simulink model "Takeoff_Sim"  (R2023a)
settings: Solver=VariableStepAuto  StartTime=0.0  StopTime=35  RelTol=1e-3
values from neighbouring files (symbols this model uses):
  AoA = 5    [initialize.m]
  AR = 6.4897    [initialize.m]
  f = 6.271    [initialize.m]
  S = 174    [initialize.m]
  Weight = 2518    [initialize.m]
undefined symbols (not defined in the file or in its folder): Accelerometer, Accelerometerdeland, Earth, Gyroscope, Gyroscopedeland, Location, Locationdeland, WGS84
libraries: simulink_extras x10, aerolibtransform2 x4, simulink x4, aerolibatmos2 x2
(part 1 of 2)
settings Model: Creator=NAILSK  LastModifiedBy=kaleb
settings RTWCC: GPUComputeCapability=5.0

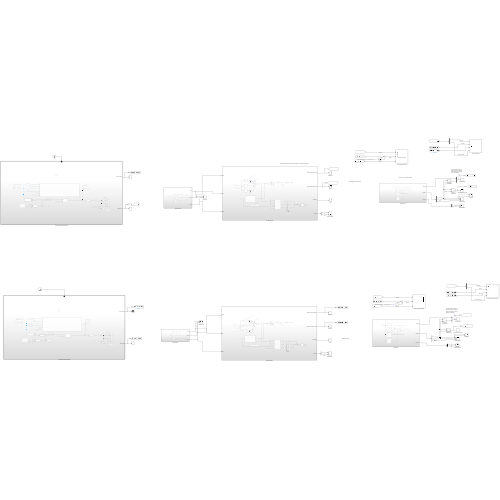
[thumbnail: Simulink's stored preview of the top-level diagram]
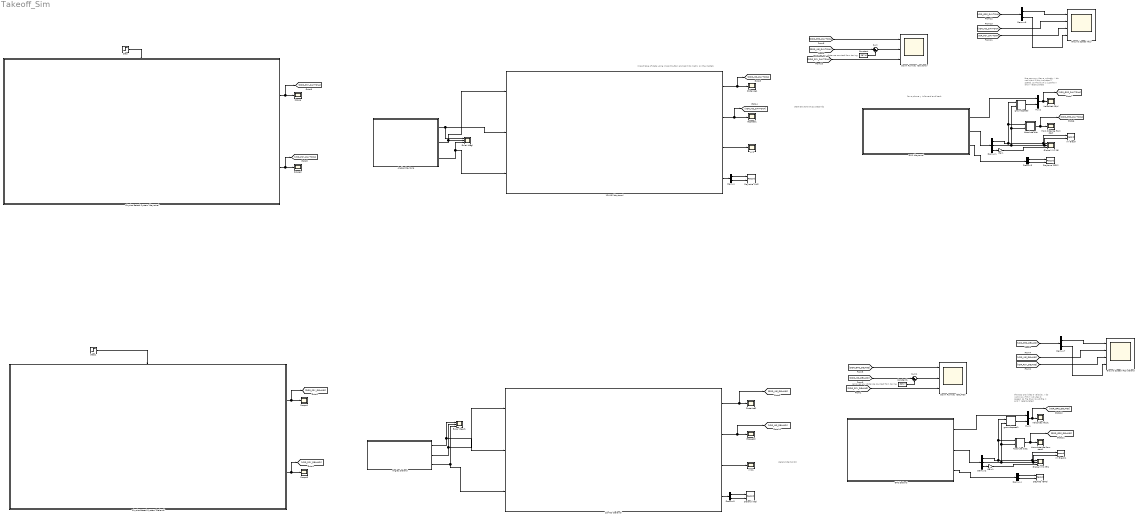
== system Takeoff_Sim ==
  note: removes any distance counted from taxing
  note: deland start at 20
  note: Start Daytona at 22 Seconds
  note: the app provides a velocity, I do not know if this includes Z speed, so the blue is just the X and Y recalculated
  note: for a phone y is foward and back
  note: import take of data using import button and set it to matrix on the matlab
  note: the app provides a velocity, I do not know if this includes Z speed, so the blue is just the X and Y recalculated
  note: removes any distance counted from taxing
  1D-INS (Deland) : Subsystem
  1D-INS (daytona) : Subsystem
  Absolute dist : Subsystem
  Absolute dist1 : Subsystem
  Angles Daytona : Subsystem
  Angles Deland : Subsystem
  Constant : Constant  Value=287.6
  Constant1 : Constant  Value=509.7
  DELAND (GPS) : Record  FileSettingsInternal="{\"entries\":[{\"content\":{\"excelSettings\":{\"content\":{},\"type\":\"Streamout.ExcelSettings\"}},\"type\":\"Streamout.FileSettingStorage\",\"uuid\":\"\"}],\"packageUris\":[\"http:\\/\\/schema.mathworks.com\\/mf0\\/streamout_blocks\\/R2020a\"],\"version\":\"1.0\"}"  Layout=[1 1]  SignalsInternal="{\"entries\":[{\"content\":{\"signals\":[{\"content\":{\"blockPath\":[],\"dimensions\":[1],\"domain\":\"\",\"lineColor\":\"#77ac30\",\"plots\":[1],\"port\":1,\"sid\":[\"\"],\"signalID\":63633,\"signalName\":\"Lat\"},\"type\":\"RecordBlkView.Signal\",\"uuid\":\"\"},{\"content\":{\"blockPath\":[],\"dimensions\":[1],\"domain\":\"\",\"lineColor\":\"#4dbeee\",\"plots\":[1],\"port\":2,\"sid\":[\"\"],\"signalID\":63637,\"signalName\":\"Long\"},\"type\":\"RecordBlkView.Signal\",\"uuid\":\"\"}]},\"type\":\"RecordBlkView.InputSignals\",\"uuid\":\"\"}],\"packageUris\":[\"http:\\/\\/schema.mathworks.com\\/mf0\\/streamout_blocks\\/R2020a\"],\"version\":\"1.0\"}"  VisualizationBindings="{\"mapsplugin\":{\"info\":[{\"bindingParametersList\":[{\"parameter\":\"Latitude\",\"signalID\":63633,\"signalName\":\"Lat\"},{\"parameter\":\"Longitude\",\"signalID\":63637,\"signalName\":\"Long\"}],\"subplotID\":1}]}}"  CompatibilityTag=XY
  Daytona (GPS) : Record  FileSettingsInternal="{\"entries\":[{\"content\":{\"excelSettings\":{\"content\":{},\"type\":\"Streamout.ExcelSettings\"}},\"type\":\"Streamout.FileSettingStorage\",\"uuid\":\"\"}],\"packageUris\":[\"http:\\/\\/schema.mathworks.com\\/mf0\\/streamout_blocks\\/R2020a\"],\"version\":\"1.0\"}"  Layout=[1 1]  SignalsInternal="{\"entries\":[{\"content\":{\"signals\":[{\"content\":{\"blockPath\":[],\"dimensions\":[1],\"domain\":\"\",\"lineColor\":\"#0072bd\",\"plots\":[1],\"port\":1,\"sid\":[\"\"],\"signalID\":63657,\"signalName\":\"Lat\"},\"type\":\"RecordBlkView.Signal\",\"uuid\":\"\"},{\"content\":{\"blockPath\":[],\"dimensions\":[1],\"domain\":\"\",\"lineColor\":\"#d95319\",\"plots\":[1],\"port\":2,\"sid\":[\"\"],\"signalID\":63661,\"signalName\":\"Long\"},\"type\":\"RecordBlkView.Signal\",\"uuid\":\"\"}]},\"type\":\"RecordBlkView.InputSignals\",\"uuid\":\"\"}],\"packageUris\":[\"http:\\/\\/schema.mathworks.com\\/mf0\\/streamout_blocks\\/R2020a\"],\"version\":\"1.0\"}"  VisualizationBindings="{\"mapsplugin\":{\"info\":[{\"bindingParametersList\":[{\"parameter\":\"Latitude\",\"signalID\":63657,\"signalName\":\"Lat\"},{\"parameter\":\"Longitude\",\"signalID\":63661,\"signalName\":\"Long\"}],\"subplotID\":1}]}}"  CompatibilityTag=XY
  Daytona (INS) : Record  FileSettingsInternal="{\"entries\":[{\"content\":{\"excelSettings\":{\"content\":{},\"type\":\"Streamout.ExcelSettings\"}},\"type\":\"Streamout.FileSettingStorage\",\"uuid\":\"\"}],\"packageUris\":[\"http:\\/\\/schema.mathworks.com\\/mf0\\/streamout_blocks\\/R2020a\"],\"version\":\"1.0\"}"  Layout=[1 1]  SignalsInternal="{\"entries\":[{\"content\":{\"signals\":[{\"content\":{\"blockPath\":[],\"dimensions\":[1],\"domain\":\"\",\"lineColor\":\"#a2142f\",\"plots\":[1],\"port\":1,\"sid\":[\"\"],\"signalID\":63665,\"signalName\":\"Lat\"},\"type\":\"RecordBlkView.Signal\",\"uuid\":\"\"},{\"content\":{\"blockPath\":[],\"dimensions\":[1],\"domain\":\"\",\"lineColor\":\"#139fff\",\"plots\":[1],\"port\":2,\"sid\":[\"\"],\"signalID\":63669,\"signalName\":\"Long\"},\"type\":\"RecordBlkView.Signal\",\"uuid\":\"\"}]},\"type\":\"RecordBlkView.InputSignals\",\"uuid\":\"\"}],\"packageUris\":[\"http:\\/\\/schema.mathworks.com\\/mf0\\/streamout_blocks\\/R2020a\"],\"version\":\"1.0\"}"  VisualizationBindings="{\"mapsplugin\":{\"info\":[{\"bindingParametersList\":[{\"parameter\":\"Latitude\",\"signalID\":63665,\"signalName\":\"Lat\"},{\"parameter\":\"Longitude\",\"signalID\":63669,\"signalName\":\"Long\"}],\"subplotID\":1}]}}"  CompatibilityTag=XY
  Deland (INS) : Record  FileSettingsInternal="{\"entries\":[{\"content\":{\"excelSettings\":{\"content\":{},\"type\":\"Streamout.ExcelSettings\"}},\"type\":\"Streamout.FileSettingStorage\",\"uuid\":\"\"}],\"packageUris\":[\"http:\\/\\/schema.mathworks.com\\/mf0\\/streamout_blocks\\/R2020a\"],\"version\":\"1.0\"}"  Layout=[1 1]  SignalsInternal="{\"entries\":[{\"content\":{\"signals\":[{\"content\":{\"blockPath\":[],\"dimensions\":[1],\"domain\":\"\",\"lineColor\":\"#ff6929\",\"plots\":[1],\"port\":1,\"sid\":[\"\"],\"signalID\":63641,\"signalName\":\"Lat\"},\"type\":\"RecordBlkView.Signal\",\"uuid\":\"\"},{\"content\":{\"blockPath\":[],\"dimensions\":[1],\"domain\":\"\",\"lineColor\":\"#b746ff\",\"plots\":[1],\"port\":2,\"sid\":[\"\"],\"signalID\":63645,\"signalName\":\"Long\"},\"type\":\"RecordBlkView.Signal\",\"uuid\":\"\"}]},\"type\":\"RecordBlkView.InputSignals\",\"uuid\":\"\"}],\"packageUris\":[\"http:\\/\\/schema.mathworks.com\\/mf0\\/streamout_blocks\\/R2020a\"],\"version\":\"1.0\"}"  VisualizationBindings="{\"mapsplugin\":{\"info\":[{\"bindingParametersList\":[{\"parameter\":\"Latitude\",\"signalID\":63641,\"signalName\":\"Lat\"},{\"parameter\":\"Longitude\",\"signalID\":63645,\"signalName\":\"Long\"}],\"subplotID\":1}]}}"  CompatibilityTag=XY
  Demux{,3..7} (6 alike) : Demux  Outputs=2
  Demux1 : Demux  Outputs=3
  Demux2 : Demux  Outputs=3
  Distance1 : Scope
  Distance2 : Scope
  Down Runway (DELAND) : Scope  NumInputPorts=3
  Down Runway (Daytona) : Scope  NumInputPorts=3
  Euler (deg) : Scope  NumInputPorts=3
  Euler (deg)1 : Scope  NumInputPorts=3
  GPS (daytona) : Subsystem
  GPS Deland : Subsystem
  Gain : Gain  Gain=-1
  Gain1 : Gain  Gain=-1
  Global XYZ (ft) : Scope  NumInputPorts=3
  Global XYZ (ft)1 : Scope  NumInputPorts=3
  Ground Speed (ft/s) : Scope  NumInputPorts=4
  Ground Speed (ft/s) deland : Scope  NumInputPorts=4
  Gspeed1 : Scope
  Gspeed2 : Scope
  Horz distance from start : Scope
  Horz distance from start1 : Scope
  Mux1 : Mux  Inputs=2
  Mux2 : Mux  Inputs=2
  Physics Based System (Deland) : Subsystem  TreatAsAtomicUnit=on
  Physics Based System (daytona) : Subsystem  TreatAsAtomicUnit=on
  Scope{,1..3} (4 alike) : Scope
  Step : Step  Time=22  SampleTime=0
  Step1 : Step  Time=20  SampleTime=0
  Sum : Sum  Inputs=|+-
  Sum1 : Sum  Inputs=|+-
  Velocities (ft/s) : Scope
  Velocities (ft/s)1 : Scope
  XY Graph : Record  FileSettingsInternal="{\"entries\":[{\"content\":{\"excelSettings\":{\"content\":{},\"type\":\"Streamout.ExcelSettings\"}},\"type\":\"Streamout.FileSettingStorage\",\"uuid\":\"\"}],\"packageUris\":[\"http:\\/\\/schema.mathworks.com\\/mf0\\/streamout_blocks\\/R2020a\"],\"version\":\"1.0\"}"  Layout=[1 1]  SignalsInternal="{\"entries\":[{\"content\":{\"signals\":[{\"content\":{\"blockPath\":[],\"dimensions\":[1],\"domain\":\"\",\"lineColor\":\"#a2142f\",\"plots\":[1],\"port\":1,\"sid\":[\"\"],\"signalID\":63673,\"signalName\":\"x\"},\"type\":\"RecordBlkView.Signal\",\"uuid\":\"\"},{\"content\":{\"blockPath\":[],\"dimensions\":[1],\"domain\":\"\",\"lineColor\":\"#139fff\",\"plots\":[1],\"port\":2,\"sid\":[\"\"],\"signalID\":63677,\"signalName\":\"y\"},\"type\":\"RecordBlkView.Signal\",\"uuid\":\"\"}]},\"type\":\"RecordBlkView.InputSignals\",\"uuid\":\"\"}],\"packageUris\":[\"http:\\/\\/schema.mathworks.com\\/mf0\\/streamout_blocks\\/R2020a\"],\"version\":\"1.0\"}"  VisualizationBindings="{\"xyplotplugin\":{\"info\":[{\"series\":[{\"bindingParametersList\":[{\"parameter\":\"X-Axis\",\"signalID\":63673,\"signalName\":\"x\"},{\"parameter\":\"Y-Axis\",\"signalID\":63677,\"signalName\":\"y\"}],\"seriesID\":32496}],\"subplotID\":1}]}}"  CompatibilityTag=XY
  XY Graph1 : Record  FileSettingsInternal="{\"entries\":[{\"content\":{\"excelSettings\":{\"content\":{},\"type\":\"Streamout.ExcelSettings\"}},\"type\":\"Streamout.FileSettingStorage\",\"uuid\":\"\"}],\"packageUris\":[\"http:\\/\\/schema.mathworks.com\\/mf0\\/streamout_blocks\\/R2020a\"],\"version\":\"1.0\"}"  Layout=[1 1]  SignalsInternal="{\"entries\":[{\"content\":{\"signals\":[{\"content\":{\"blockPath\":[],\"dimensions\":[1],\"domain\":\"\",\"lineColor\":\"#a2142f\",\"plots\":[1],\"port\":1,\"sid\":[\"\"],\"signalID\":63649,\"signalName\":\"x\"},\"type\":\"RecordBlkView.Signal\",\"uuid\":\"\"},{\"content\":{\"blockPath\":[],\"dimensions\":[1],\"domain\":\"\",\"lineColor\":\"#139fff\",\"plots\":[1],\"port\":2,\"sid\":[\"\"],\"signalID\":63653,\"signalName\":\"y\"},\"type\":\"RecordBlkView.Signal\",\"uuid\":\"\"}]},\"type\":\"RecordBlkView.InputSignals\",\"uuid\":\"\"}],\"packageUris\":[\"http:\\/\\/schema.mathworks.com\\/mf0\\/streamout_blocks\\/R2020a\"],\"version\":\"1.0\"}"  VisualizationBindings="{\"xyplotplugin\":{\"info\":[{\"series\":[{\"bindingParametersList\":[{\"parameter\":\"X-Axis\",\"signalID\":63649,\"signalName\":\"x\"},{\"parameter\":\"Y-Axis\",\"signalID\":63653,\"signalName\":\"y\"}],\"seriesID\":5620}],\"subplotID\":1}]}}"  CompatibilityTag=XY
  XYZ : Scope
  XYZ1 : Scope
  groundspeed : Subsystem
  groundspeed1 : Subsystem
  wires:
  1D-INS (daytona)/1(Distance Down Runway (ft)) -> [DDR_INS_DAYTONA], Distance1/1
  1D-INS (daytona)/2(Velocity Down Runway (ft/s)) -> [VDR_INS_DAYTONA], Gspeed1/1
  GPS (daytona)/1(velocity) -> Mux2/1
  GPS (daytona)/2(Distance) -> Demux1/1
  Demux1/1 -> Absolute dist/1(x), groundspeed/1(x), XY Graph/1, Global XYZ (ft)/1  "x"
  Demux1/2 -> Absolute dist/2(y), groundspeed/2(y), XY Graph/2, Global XYZ (ft)/2  "y"
  Demux1/3 -> Gain/1  "z"
  Gain/1 -> Global XYZ (ft)/3
  groundspeed/1(Out1) -> Mux2/2
  Mux2/1 -> [VDR_GPS_DAYTONA], Velocities (ft/s)/1
  Angles Daytona/1(roll1) -> 1D-INS (daytona)/2(roll), Euler (deg)/1
  Angles Daytona/2(pitch1) -> 1D-INS (daytona)/1(pitch), Euler (deg)/2
  Angles Daytona/3(yaw1) -> 1D-INS (daytona)/3(yaw), Euler (deg)/3
  Absolute dist/1(Out1) -> [DDR_GPS_DAYTONA], Horz distance from start/1
  1D-INS (daytona)/3(Global (ft/s)) -> XYZ/1
  1D-INS (daytona)/4(Lat/Long) -> Demux/1
  Demux/1 -> Daytona (INS)/1  "Lat"
  Demux/2 -> Daytona (INS)/2  "Long"
  Demux3/1 -> Daytona (GPS)/1  "Lat"
  Demux3/2 -> Daytona (GPS)/2  "Long"
  GPS (daytona)/3(Lat/Long) -> Demux3/1
  Demux5/2 -> Deland (INS)/2  "Long"
  1D-INS (Deland)/3(Global (ft/s)) -> XYZ1/1
  Demux5/1 -> Deland (INS)/1  "Lat"
  1D-INS (Deland)/4(Lat/Long) -> Demux5/1
  1D-INS (Deland)/2(Velocity Down Runway (ft/s)) -> [VDR_INS_DELAND], Gspeed2/1
  1D-INS (Deland)/1(Distance Down Runway (ft)) -> [DDR_INS_DELAND], Distance2/1
  Angles Deland/3(yaw1) -> 1D-INS (Deland)/3(yaw), Euler (deg)1/3
  Angles Deland/2(pitch1) -> Euler (deg)1/2, 1D-INS (Deland)/1(pitch)
  Angles Deland/1(roll1) -> Euler (deg)1/1, 1D-INS (Deland)/2(roll)
  Step/1 -> Physics Based System (daytona)/Enable
  Physics Based System (daytona)/2(Velocity (ft/s)) -> [VDR_PSY_DAYTONA], Scope2/1
  Physics Based System (daytona)/1(Ft down runway) -> [DDR_PSY_DAYTONA], Scope/1
  [DDR_GPS_DAYTONA] -> Down Runway (Daytona)/1  "GPS (ft)"
  [DDR_INS_DAYTONA] -> Sum/1  "INS (ft)"
  [DDR_PSY_DAYTONA] -> Down Runway (Daytona)/3  "PSY (ft)"
  Constant/1 -> Sum/2
  Sum/1 -> Down Runway (Daytona)/2  "INS (ft)"
  [VDR_PSY_DAYTONA] -> Ground Speed (ft/s)/3  "PSY (ft/s)"
  [VDR_INS_DAYTONA] -> Ground Speed (ft/s)/2  "INS (ft/s)"
  [VDR_GPS_DAYTONA] -> Demux6/1
  Demux6/2 -> Ground Speed (ft/s)/4  "Derived GPS (ft/s)"
  Demux6/1 -> Ground Speed (ft/s)/1  "GPS (ft/s)"
  Physics Based System (Deland)/1(Ft down runway) -> Scope1/1, [DDR_PSY_DELAND]
  Physics Based System (Deland)/2(Velocity (ft/s)) -> Scope3/1, [VDR_PSY_DELAND]
  Step1/1 -> Physics Based System (Deland)/Enable
  groundspeed1/1(Out1) -> Mux1/2
  Absolute dist1/1(Out1) -> [DDR_GPS_DELAND], Horz distance from start1/1
  Demux4/2 -> DELAND (GPS)/2  "Long"
  GPS Deland/1(velocity) -> Mux1/1
  Gain1/1 -> Global XYZ (ft)1/3
  GPS Deland/3(Lat/Long) -> Demux4/1
  Demux2/1 -> Absolute dist1/1(x), groundspeed1/1(x), XY Graph1/1, Global XYZ (ft)1/1  "x"
  GPS Deland/2(Distance) -> Demux2/1
  Demux2/3 -> Gain1/1  "z"
  Demux4/1 -> DELAND (GPS)/1  "Lat"
  Mux1/1 -> [VDR_GPS_DELAND], Velocities (ft/s)1/1
  Demux2/2 -> Absolute dist1/2(y), groundspeed1/2(y), XY Graph1/2, Global XYZ (ft)1/2  "y"
  Demux7/1 -> Ground Speed (ft/s) deland/1  "GPS (ft/s)"
  Demux7/2 -> Ground Speed (ft/s) deland/4  "Derived GPS (ft/s)"
  [VDR_GPS_DELAND] -> Demux7/1
  [VDR_INS_DELAND] -> Ground Speed (ft/s) deland/2  "INS (ft/s)"
  [VDR_PSY_DELAND] -> Ground Speed (ft/s) deland/3  "PSY (ft/s)"
  Sum1/1 -> Down Runway (DELAND)/2  "INS (ft)"
  Constant1/1 -> Sum1/2
  [DDR_PSY_DELAND] -> Down Runway (DELAND)/3  "PSY (ft)"
  [DDR_INS_DELAND] -> Sum1/1  "INS (ft)"
  [DDR_GPS_DELAND] -> Down Runway (DELAND)/1  "GPS (ft)"

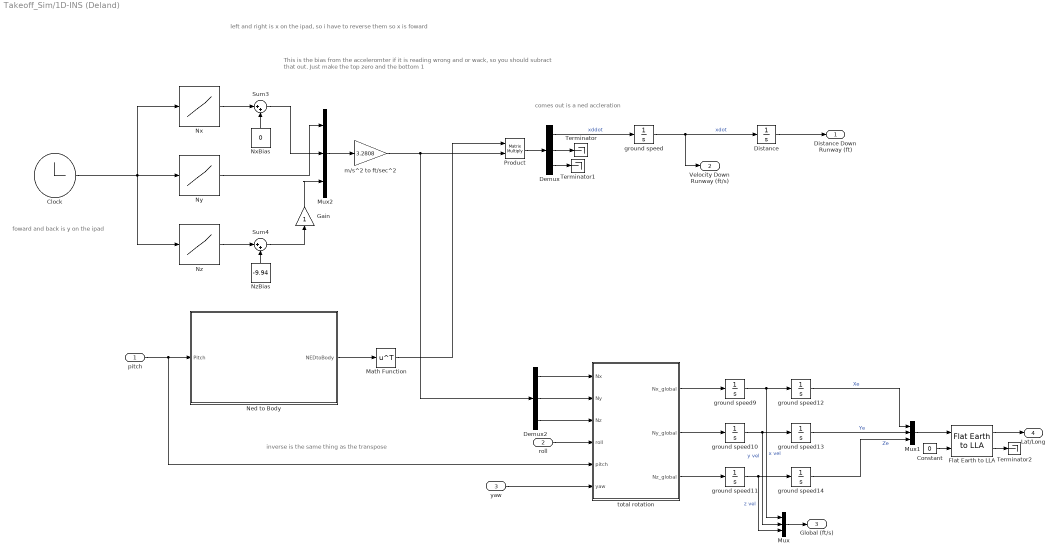
== system Takeoff_Sim/1D-INS (Deland) ==
  note: foward and back is y on the ipad
  note: left and right is x on the ipad, so i have to reverse them so x is foward
  note: This is the bias from the acceleromter if it is reading wrong and or wack, so you should subract that out. Just make the top zero and the bottom 1
  note: inverse is the same thing as the transpose
  note: comes out is a ned accleration
  pitch : Inport
  roll : Inport  Port=2
  yaw : Inport  Port=3
  Clock : Clock
  Constant : Constant  Value=0
  Demux : Demux  Outputs=3
  Demux2 : Demux  Outputs=3
  Distance : Integrator
  Flat Earth to LLA : aerolibtransform2/Flat Earth to LLA  units=English  ptype=Earth (WGS84)  F=1/298.257223563  R=20925646.3255  refPosPort=off  LL0=[2.906098674E1 -8.128727349E1]  psi=0
  Gain : Gain
  Math Function : Math  Operator=transpose
  Mux : Mux  Inputs=3
  Mux1 : Mux  Inputs=3
  Mux2 : Mux  Inputs=3
  Ned to Body : Subsystem
  Nx : Lookup_n-D  NumberOfTableDimensions=1  BreakpointsForDimension1=Accelerometerdeland(:,1)  Table=Accelerometerdeland(:,2)  InternalRulePriority=Speed  RndMeth=Simplest
  NxBias : Constant  Value=0
  Ny : Lookup_n-D  NumberOfTableDimensions=1  BreakpointsForDimension1=Accelerometerdeland(:,1)  Table=Accelerometerdeland(:,3)  InternalRulePriority=Speed  RndMeth=Simplest
  Nz : Lookup_n-D  NumberOfTableDimensions=1  BreakpointsForDimension1=Accelerometerdeland(:,1)  Table=Accelerometerdeland(:,4)  InternalRulePriority=Speed  RndMeth=Simplest
  NzBias : Constant  Value=-9.94
  Product : Product  Multiplication=Matrix(*)
  Sum3 : Sum  Inputs=|++
  Sum4 : Sum  Inputs=|++
  Terminator : Terminator
  Terminator1 : Terminator
  Terminator2 : Terminator
  ground speed : Integrator  InitialCondition=8.55
  ground speed{9..14} (6 alike) : Integrator
  m/s^2 to ft/sec^2 : Gain  Gain=3.2808
  total rotation : MATLAB Function  TreatAsAtomicUnit=on
  Distance Down Runway (ft) : Outport
  Velocity Down Runway (ft/s) : Outport  Port=2
  Global (ft/s) : Outport  Port=3
  Lat/Long : Outport  Port=4
  wires:
  Sum3/1 -> Mux2/2
  Product/1 -> Demux/1
  Ned to Body/1(NEDtoBody) -> Math Function/1
  Nz/1 -> Sum4/1
  Clock/1 -> Nx/1, Nz/1, Ny/1
  Mux2/1 -> m/s^2 to ft/sec^2/1
  NxBias/1 -> Sum3/2
  Nx/1 -> Sum3/1
  NzBias/1 -> Sum4/2
  m/s^2 to ft/sec^2/1 -> Demux2/1, Product/2
  Demux/1 -> ground speed/1  "xddot"
  Math Function/1 -> Product/1
  ground speed/1 -> Distance/1, Velocity Down Runway (ft/s)/1  "xdot"
  Ny/1 -> Mux2/1
  Sum4/1 -> Gain/1
  Distance/1 -> Distance Down Runway (ft)/1
  pitch/1 -> total rotation/5(pitch), Ned to Body/1(Pitch)
  Demux2/1 -> total rotation/1(Nx)
  Demux2/2 -> total rotation/2(Ny)
  Demux2/3 -> total rotation/3(Nz)
  roll/1 -> total rotation/4(roll)
  ground speed14/1 -> Mux1/3  "Ze"
  ground speed13/1 -> Mux1/2  "Ye"
  ground speed12/1 -> Mux1/1  "Xe"
  ground speed11/1 -> Mux/3, ground speed14/1  "z vel"
  ground speed10/1 -> Mux/2, ground speed13/1  "y vel"
  ground speed9/1 -> Mux/1, ground speed12/1  "x vel"
  total rotation/3(Nz_global) -> ground speed11/1
  total rotation/2(Ny_global) -> ground speed10/1
  total rotation/1(Nx_global) -> ground speed9/1
  Demux/2 -> Terminator/1
  Demux/3 -> Terminator1/1
  Mux/1 -> Global (ft/s)/1
  Constant/1 -> Flat Earth to LLA/2
  Flat Earth to LLA/2 -> Terminator2/1
  Mux1/1 -> Flat Earth to LLA/1
  Flat Earth to LLA/1 -> Lat/Long/1
  yaw/1 -> total rotation/6(yaw)
  Gain/1 -> Mux2/3

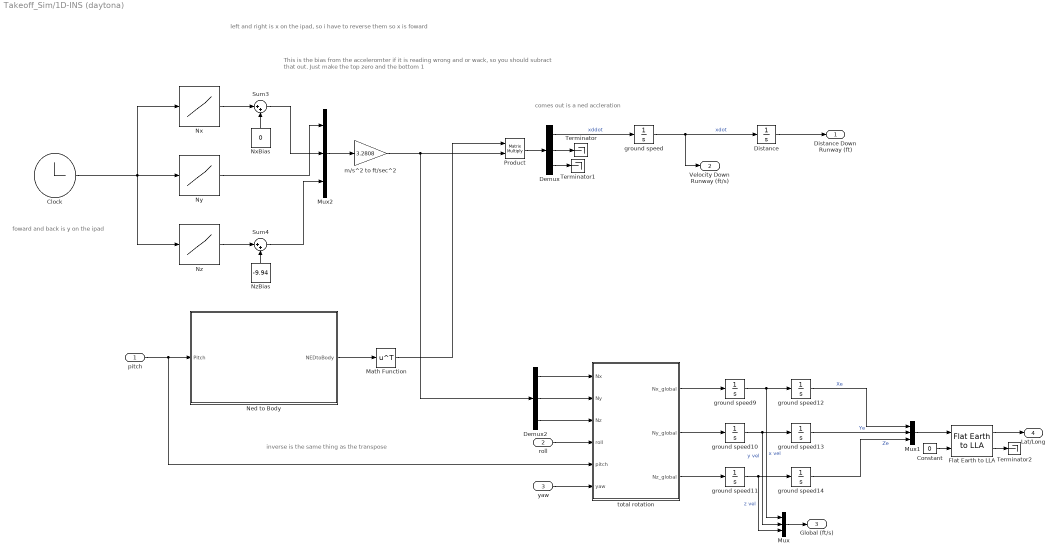
== system Takeoff_Sim/1D-INS (daytona) ==
  note: foward and back is y on the ipad
  note: left and right is x on the ipad, so i have to reverse them so x is foward
  note: This is the bias from the acceleromter if it is reading wrong and or wack, so you should subract that out. Just make the top zero and the bottom 1
  note: inverse is the same thing as the transpose
  note: comes out is a ned accleration
  pitch : Inport
  roll : Inport  Port=2
  yaw : Inport  Port=3
  Clock : Clock
  Constant : Constant  Value=0
  Demux : Demux  Outputs=3
  Demux2 : Demux  Outputs=3
  Distance : Integrator
  Flat Earth to LLA : aerolibtransform2/Flat Earth to LLA  units=English  ptype=Earth (WGS84)  F=1/298.257223563  R=20925646.3255  refPosPort=off  LL0=[2.917987119E1 -8.106194666E1]  psi=0
  Math Function : Math  Operator=transpose
  Mux : Mux  Inputs=3
  Mux1 : Mux  Inputs=3
  Mux2 : Mux  Inputs=3
  Ned to Body : Subsystem
  Nx : Lookup_n-D  NumberOfTableDimensions=1  BreakpointsForDimension1=Accelerometer(:,1)  Table=Accelerometer(:,2)  InternalRulePriority=Speed  RndMeth=Simplest
  NxBias : Constant  Value=0
  Ny : Lookup_n-D  NumberOfTableDimensions=1  BreakpointsForDimension1=Accelerometer(:,1)  Table=Accelerometer(:,3)  InternalRulePriority=Speed  RndMeth=Simplest
  Nz : Lookup_n-D  NumberOfTableDimensions=1  BreakpointsForDimension1=Accelerometer(:,1)  Table=Accelerometer(:,4)  InternalRulePriority=Speed  RndMeth=Simplest
  NzBias : Constant  Value=-9.94
  Product : Product  Multiplication=Matrix(*)
  Sum3 : Sum  Inputs=|++
  Sum4 : Sum  Inputs=|++
  Terminator : Terminator
  Terminator1 : Terminator
  Terminator2 : Terminator
  ground speed{,9..14} (7 alike) : Integrator
  m/s^2 to ft/sec^2 : Gain  Gain=3.2808
  total rotation : MATLAB Function  TreatAsAtomicUnit=on
  Distance Down Runway (ft) : Outport
  Velocity Down Runway (ft/s) : Outport  Port=2
  Global (ft/s) : Outport  Port=3
  Lat/Long : Outport  Port=4
  wires:
  Sum3/1 -> Mux2/2
  Product/1 -> Demux/1
  Ned to Body/1(NEDtoBody) -> Math Function/1
  Nz/1 -> Sum4/1
  Clock/1 -> Nx/1, Nz/1, Ny/1
  Mux2/1 -> m/s^2 to ft/sec^2/1
  NxBias/1 -> Sum3/2
  Nx/1 -> Sum3/1
  NzBias/1 -> Sum4/2
  m/s^2 to ft/sec^2/1 -> Demux2/1, Product/2
  Demux/1 -> ground speed/1  "xddot"
  Math Function/1 -> Product/1
  ground speed/1 -> Distance/1, Velocity Down Runway (ft/s)/1  "xdot"
  Ny/1 -> Mux2/1
  Sum4/1 -> Mux2/3
  Distance/1 -> Distance Down Runway (ft)/1
  pitch/1 -> total rotation/5(pitch), Ned to Body/1(Pitch)
  Demux2/1 -> total rotation/1(Nx)
  Demux2/2 -> total rotation/2(Ny)
  Demux2/3 -> total rotation/3(Nz)
  yaw/1 -> total rotation/6(yaw)
  roll/1 -> total rotation/4(roll)
  ground speed14/1 -> Mux1/3  "Ze"
  ground speed13/1 -> Mux1/2  "Ye"
  ground speed12/1 -> Mux1/1  "Xe"
  ground speed11/1 -> Mux/3, ground speed14/1  "z vel"
  ground speed10/1 -> Mux/2, ground speed13/1  "y vel"
  ground speed9/1 -> Mux/1, ground speed12/1  "x vel"
  total rotation/3(Nz_global) -> ground speed11/1
  total rotation/2(Ny_global) -> ground speed10/1
  total rotation/1(Nx_global) -> ground speed9/1
  Demux/2 -> Terminator/1
  Demux/3 -> Terminator1/1
  Mux/1 -> Global (ft/s)/1
  Constant/1 -> Flat Earth to LLA/2
  Flat Earth to LLA/2 -> Terminator2/1
  Mux1/1 -> Flat Earth to LLA/1
  Flat Earth to LLA/1 -> Lat/Long/1

== system Takeoff_Sim/Absolute dist ==
  note: since this is GPS, i cannot measure from the start, i geo synced this position with a time. because the current data set includes some taxiing , this removes that
  x : Inport
  y : Inport  Port=2
  Abs : Abs  SaturateOnIntegerOverflow=off
  Abs1 : Abs  SaturateOnIntegerOverflow=off
  Start Posx : Constant  Value=-210.4
  Sum : Sum  Inputs=|-+
  Sum1 : Sum  Inputs=|-+
  Sum4 : Sum  Inputs=|++
  start pos y : Constant  Value=164.6
  Out1 : Outport
  wires:
  y/1 -> Sum1/2
  Abs/1 -> Sum4/1
  x/1 -> Sum/2
  Abs1/1 -> Sum4/2
  Sum4/1 -> Out1/1
  Start Posx/1 -> Sum/1
  Sum/1 -> Abs/1
  start pos y/1 -> Sum1/1
  Sum1/1 -> Abs1/1

== system Takeoff_Sim/Absolute dist1 ==
  note: since this is GPS, i cannot measure from the start, i geo synced this position with a time. because the current data set includes some taxiing , this removes that
  x : Inport
  y : Inport  Port=2
  Abs : Abs  SaturateOnIntegerOverflow=off
  Abs1 : Abs  SaturateOnIntegerOverflow=off
  Start Posx : Constant  Value=84.1
  Sum : Sum  Inputs=|-+
  Sum1 : Sum  Inputs=|-+
  Sum4 : Sum  Inputs=|++
  start pos y : Constant  Value=-134.8
  Out1 : Outport
  wires:
  y/1 -> Sum1/2
  Abs/1 -> Sum4/1
  x/1 -> Sum/2
  Abs1/1 -> Sum4/2
  Sum4/1 -> Out1/1
  Start Posx/1 -> Sum/1
  Sum/1 -> Abs/1
  start pos y/1 -> Sum1/1
  Sum1/1 -> Abs1/1

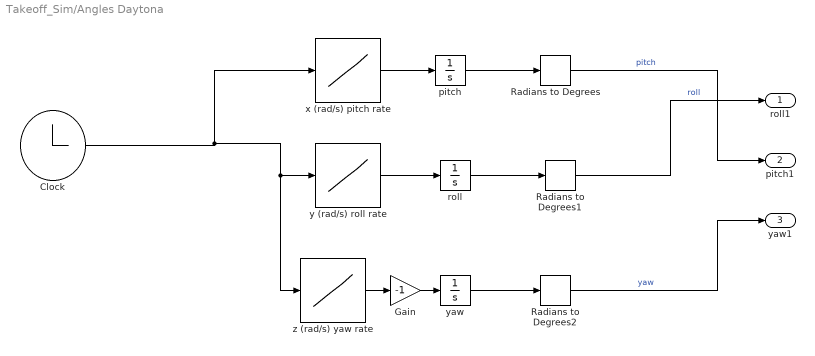
== system Takeoff_Sim/Angles Daytona ==
  Clock : Clock
  Gain : Gain  Gain=-1
  Radians to Degrees : simulink_extras/Transformations/Radians to Degrees
  Radians to Degrees1 : simulink_extras/Transformations/Radians to Degrees
  Radians to Degrees2 : simulink_extras/Transformations/Radians to Degrees
  pitch : Integrator  InitialCondition=.0995
  roll : Integrator
  x (rad/s) pitch rate : Lookup_n-D  NumberOfTableDimensions=1  BreakpointsForDimension1=Gyroscope(:,1)  Table=Gyroscope(:,2)  InternalRulePriority=Speed  RndMeth=Simplest
  y (rad/s) roll rate : Lookup_n-D  NumberOfTableDimensions=1  BreakpointsForDimension1=Gyroscope(:,1)  Table=Gyroscope(:,3)  InternalRulePriority=Speed  RndMeth=Simplest
  yaw : Integrator  InitialCondition=pi/180*165
  z (rad/s) yaw rate : Lookup_n-D  NumberOfTableDimensions=1  BreakpointsForDimension1=Gyroscope(:,1)  Table=Gyroscope(:,4)  InternalRulePriority=Speed  RndMeth=Simplest
  roll1 : Outport
  pitch1 : Outport  Port=2
  yaw1 : Outport  Port=3
  wires:
  pitch/1 -> Radians to Degrees/1
  Radians to Degrees2/1 -> yaw1/1  "yaw"
  yaw/1 -> Radians to Degrees2/1
  Clock/1 -> z (rad/s) yaw rate/1, y (rad/s) roll rate/1, x (rad/s) pitch rate/1
  y (rad/s) roll rate/1 -> roll/1
  roll/1 -> Radians to Degrees1/1
  x (rad/s) pitch rate/1 -> pitch/1
  Radians to Degrees/1 -> pitch1/1  "pitch"
  Radians to Degrees1/1 -> roll1/1  "roll"
  z (rad/s) yaw rate/1 -> Gain/1
  Gain/1 -> yaw/1

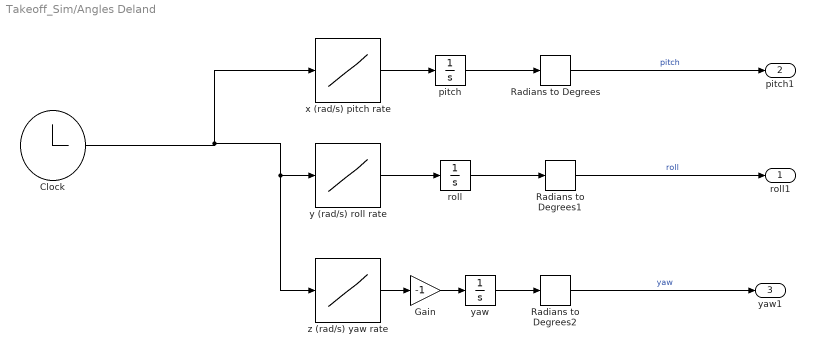
== system Takeoff_Sim/Angles Deland ==
  Clock : Clock
  Gain : Gain  Gain=-1
  Radians to Degrees : simulink_extras/Transformations/Radians to Degrees
  Radians to Degrees1 : simulink_extras/Transformations/Radians to Degrees
  Radians to Degrees2 : simulink_extras/Transformations/Radians to Degrees
  pitch : Integrator  InitialCondition=.0995
  roll : Integrator
  x (rad/s) pitch rate : Lookup_n-D  NumberOfTableDimensions=1  BreakpointsForDimension1=Gyroscopedeland(:,1)  Table=Gyroscopedeland(:,2)  InternalRulePriority=Speed  RndMeth=Simplest
  y (rad/s) roll rate : Lookup_n-D  NumberOfTableDimensions=1  BreakpointsForDimension1=Gyroscopedeland(:,1)  Table=Gyroscopedeland(:,3)  InternalRulePriority=Speed  RndMeth=Simplest
  yaw : Integrator  InitialCondition=-1.75
  z (rad/s) yaw rate : Lookup_n-D  NumberOfTableDimensions=1  BreakpointsForDimension1=Gyroscopedeland(:,1)  Table=Gyroscopedeland(:,4)  InternalRulePriority=Speed  RndMeth=Simplest
  roll1 : Outport
  pitch1 : Outport  Port=2
  yaw1 : Outport  Port=3
  wires:
  pitch/1 -> Radians to Degrees/1
  Radians to Degrees2/1 -> yaw1/1  "yaw"
  yaw/1 -> Radians to Degrees2/1
  Clock/1 -> z (rad/s) yaw rate/1, y (rad/s) roll rate/1, x (rad/s) pitch rate/1
  y (rad/s) roll rate/1 -> roll/1
  z (rad/s) yaw rate/1 -> Gain/1
  roll/1 -> Radians to Degrees1/1
  x (rad/s) pitch rate/1 -> pitch/1
  Radians to Degrees/1 -> pitch1/1  "pitch"
  Radians to Degrees1/1 -> roll1/1  "roll"
  Gain/1 -> yaw/1

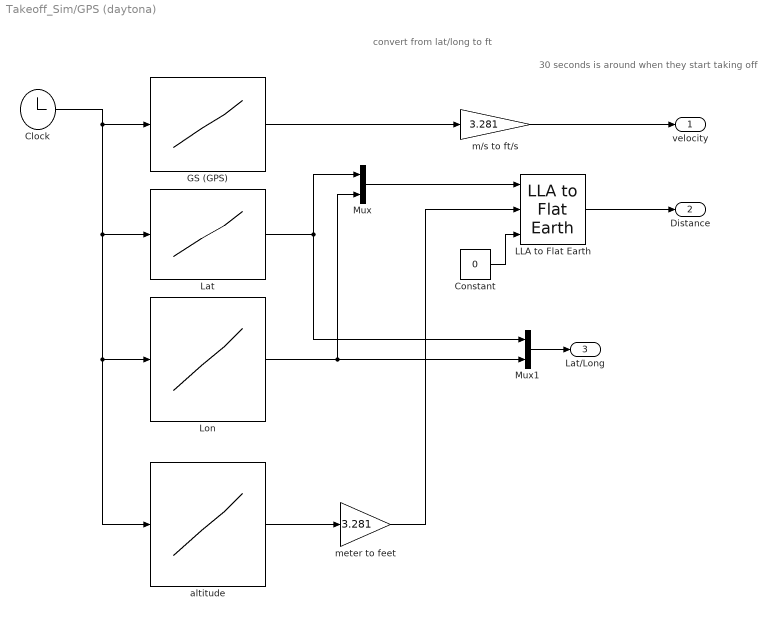
== system Takeoff_Sim/GPS (daytona) ==
  note: 30 seconds is around when they start taking off
  note: convert from lat/long to ft
  Clock : Clock
  Constant : Constant  Value=0
  GS (GPS) : Lookup_n-D  NumberOfTableDimensions=1  BreakpointsForDimension1=Location(:,1)  Table=Location(:,5)  InternalRulePriority=Speed  RndMeth=Simplest
  LLA to Flat Earth : aerolibtransform2/LLA to Flat Earth  units=English  ptype=Earth (WGS84)  F=1/298.257223563  R=20925646.3255  refPosPort=off  LL0=[2.917987119E1 -8.106194666E1]  psi=0
  Lat : Lookup_n-D  NumberOfTableDimensions=1  BreakpointsForDimension1=Location(:,1)  Table=Location(:,2)  InternalRulePriority=Speed  RndMeth=Simplest
  Lon : Lookup_n-D  NumberOfTableDimensions=1  BreakpointsForDimension1=Location(:,1)  Table=Location(:,3)  InternalRulePriority=Speed  RndMeth=Simplest
  Mux : Mux  Inputs=2
  Mux1 : Mux  Inputs=2
  altitude : Lookup_n-D  NumberOfTableDimensions=1  BreakpointsForDimension1=Location(:,1)  Table=Location(:,4)  InternalRulePriority=Speed  RndMeth=Simplest
  m/s to ft/s : Gain  Gain=3.281
  meter to feet : Gain  Gain=3.281
  velocity : Outport
  Distance : Outport  Port=2
  Lat/Long : Outport  Port=3
  wires:
  Clock/1 -> altitude/1, Lon/1, Lat/1, GS (GPS)/1
  Lat/1 -> Mux1/1, Mux/1
  Lon/1 -> Mux/2, Mux1/2
  Mux/1 -> LLA to Flat Earth/1
  GS (GPS)/1 -> m/s to ft/s/1
  m/s to ft/s/1 -> velocity/1
  Constant/1 -> LLA to Flat Earth/3
  altitude/1 -> meter to feet/1
  meter to feet/1 -> LLA to Flat Earth/2
  LLA to Flat Earth/1 -> Distance/1
  Mux1/1 -> Lat/Long/1

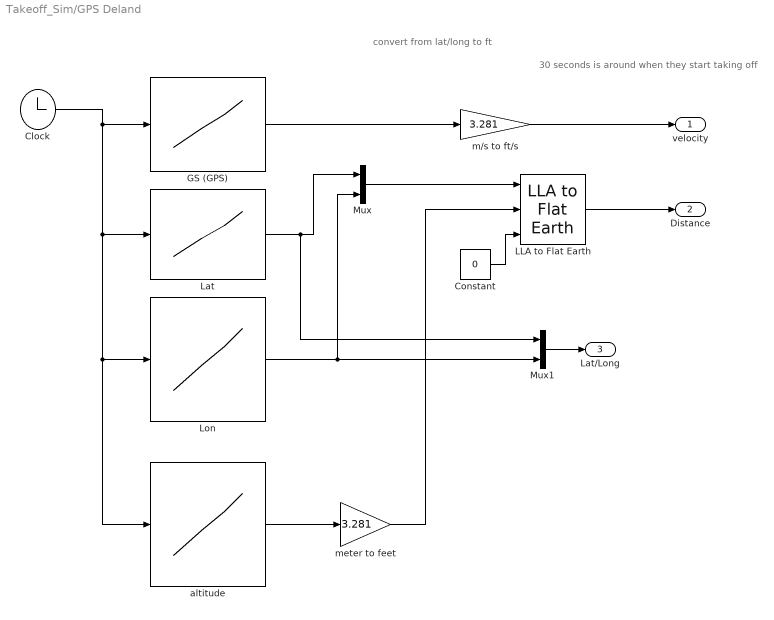
== system Takeoff_Sim/GPS Deland ==
  note: 30 seconds is around when they start taking off
  note: convert from lat/long to ft
  Clock : Clock
  Constant : Constant  Value=0
  GS (GPS) : Lookup_n-D  NumberOfTableDimensions=1  BreakpointsForDimension1=Locationdeland(:,1)  Table=Locationdeland(:,5)  InternalRulePriority=Speed  RndMeth=Simplest
  LLA to Flat Earth : aerolibtransform2/LLA to Flat Earth  units=English  ptype=Earth (WGS84)  F=1/298.257223563  R=20925646.3255  refPosPort=off  LL0=[2.906098674E1 -8.128727349E1]  psi=0
  Lat : Lookup_n-D  NumberOfTableDimensions=1  BreakpointsForDimension1=Locationdeland(:,1)  Table=Locationdeland(:,2)  InternalRulePriority=Speed  RndMeth=Simplest
  Lon : Lookup_n-D  NumberOfTableDimensions=1  BreakpointsForDimension1=Locationdeland(:,1)  Table=Locationdeland(:,3)  InternalRulePriority=Speed  RndMeth=Simplest
  Mux : Mux  Inputs=2
  Mux1 : Mux  Inputs=2
  altitude : Lookup_n-D  NumberOfTableDimensions=1  BreakpointsForDimension1=Locationdeland(:,1)  Table=Locationdeland(:,4)  InternalRulePriority=Speed  RndMeth=Simplest
  m/s to ft/s : Gain  Gain=3.281
  meter to feet : Gain  Gain=3.281
  velocity : Outport
  Distance : Outport  Port=2
  Lat/Long : Outport  Port=3
  wires:
  Clock/1 -> altitude/1, Lon/1, Lat/1, GS (GPS)/1
  Lat/1 -> Mux1/1, Mux/1
  Lon/1 -> Mux/2, Mux1/2
  Mux/1 -> LLA to Flat Earth/1
  GS (GPS)/1 -> m/s to ft/s/1
  m/s to ft/s/1 -> velocity/1
  Constant/1 -> LLA to Flat Earth/3
  altitude/1 -> meter to feet/1
  meter to feet/1 -> LLA to Flat Earth/2
  LLA to Flat Earth/1 -> Distance/1
  Mux1/1 -> Lat/Long/1

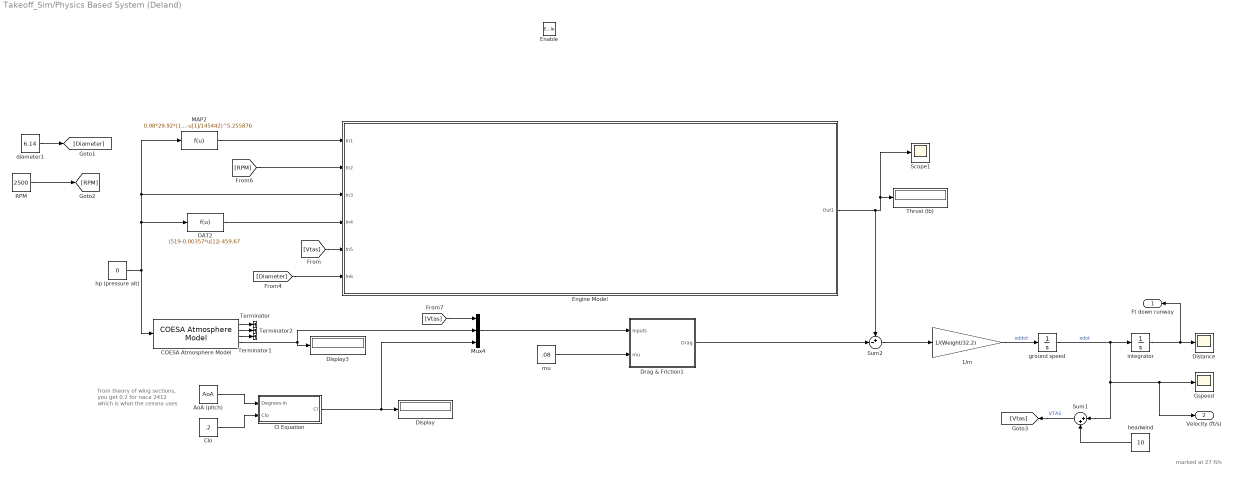
== system Takeoff_Sim/Physics Based System (Deland) ==
  note: from theory of wing sections, you get 0.2 for naca 2412 which is what the cessna uses
  note: marked at 27 ft/s
  Enable : EnablePort
  1/m : Gain  Gain=1/(Weight/32.2)
  AoA (pitch) : Constant  Value=AoA
  COESA Atmosphere Model : aerolibatmos2/COESA Atmosphere Model  units=English (Velocity in ft/s)  spec=1976 COESA-extended U.S. Standard Atmosphere  model=Profile  profile_var=High temperature  profile_percent=1%  profile_alt=5 km (16404 ft)  envelope_var=High temperature  envelope_percent=1%  action=Warning
  Cl Equation : Subsystem
  Clo : Constant  Value=.2
  Display : Display
  Display3 : Display
  Distance : Scope
  Drag & Friction1 : Subsystem  VariantControl=Choice
  Engine Model : Subsystem
  Gspeed : Scope
  MAP2 : Fcn  Expr=0.98*29.92*(1-u[1]/145442)^5.255876
  Mux4 : Mux  Inputs=3
  OAT2 : Fcn  Expr=(519-0.00357*u[1])-459.67
  RPM : Constant  Value=2500
  Scope1 : Scope
  Sum1 : Sum  Inputs=|++
  Sum2 : Sum  Inputs=+-|
  Terminator : Terminator
  Terminator1 : Terminator
  Terminator2 : Terminator
  Thrust (lb) : Display
  diameter1 : Constant  Value=6.14
  ground speed : Integrator  InitialCondition=20
  headwind : Constant  Value=10
  hp (pressure alt) : Constant  Value=0
  integrator : Integrator
  mu : Constant  Value=.08
  Ft down runway : Outport
  Velocity (ft/s) : Outport  Port=2
  wires:
  integrator/1 -> Distance/1, Ft down runway/1
  diameter1/1 -> [Diameter]
  [RPM] -> Engine Model/2(In2)
  OAT2/1 -> Engine Model/4(In4)
  COESA Atmosphere Model/4 -> Mux4/2, Display3/1
  headwind/1 -> Sum1/2
  [Diameter] -> Engine Model/6(In6)
  MAP2/1 -> Engine Model/1(In1)
  hp (pressure alt)/1 -> COESA Atmosphere Model/1, Engine Model/3(In3), MAP2/1, OAT2/1
  ground speed/1 -> integrator/1, Gspeed/1, Velocity (ft/s)/1, Sum1/1  "xdot"
  RPM/1 -> [RPM]
  Mux4/1 -> Drag & Friction1/1(Inputs)
  Cl Equation/1(Cl) -> Display/1, Mux4/3
  1/m/1 -> ground speed/1  "xddot"
  Engine Model/1(Out1) -> Sum2/1, Thrust (lb)/1, Scope1/1
  Sum2/1 -> 1/m/1
  [Vtas] -> Engine Model/5(In5)
  COESA Atmosphere Model/2 -> Terminator2/1
  COESA Atmosphere Model/1 -> Terminator/1
  COESA Atmosphere Model/3 -> Terminator1/1
  AoA (pitch)/1 -> Cl Equation/1(Degrees in)
  Sum1/1 -> [Vtas]  "VTAS"
  mu/1 -> Drag & Friction1/2(mu)
  Drag & Friction1/1(Drag) -> Sum2/2
  Clo/1 -> Cl Equation/2(Clo)
  [Vtas] -> Mux4/1

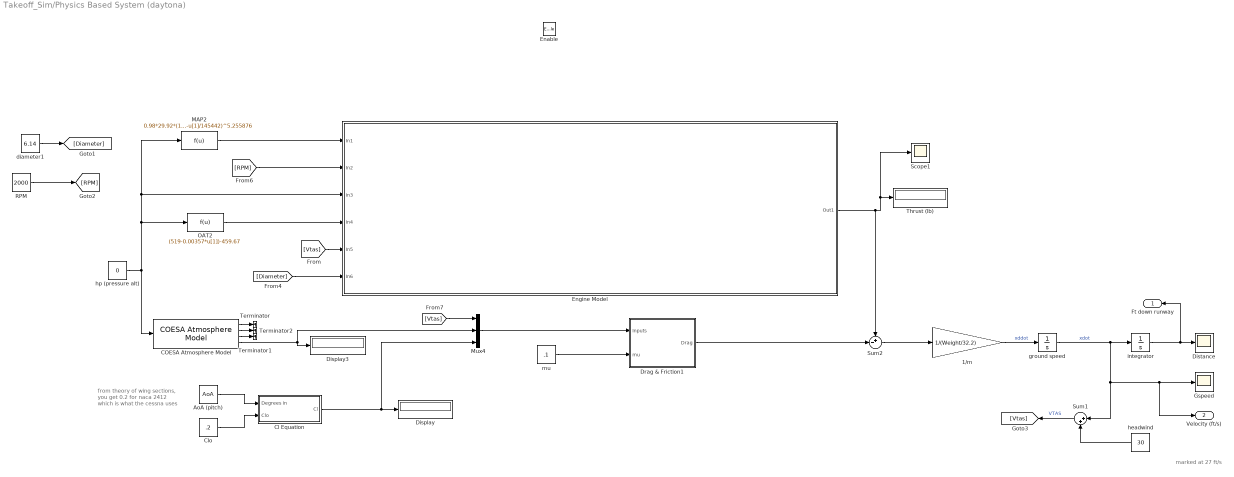
== system Takeoff_Sim/Physics Based System (daytona) ==
  note: marked at 27 ft/s
  note: from theory of wing sections, you get 0.2 for naca 2412 which is what the cessna uses
  Enable : EnablePort
  1/m : Gain  Gain=1/(Weight/32.2)
  AoA (pitch) : Constant  Value=AoA
  COESA Atmosphere Model : aerolibatmos2/COESA Atmosphere Model  units=English (Velocity in ft/s)  spec=1976 COESA-extended U.S. Standard Atmosphere  model=Profile  profile_var=High temperature  profile_percent=1%  profile_alt=5 km (16404 ft)  envelope_var=High temperature  envelope_percent=1%  action=Warning
  Cl Equation : Subsystem
  Clo : Constant  Value=.2
  Display : Display
  Display3 : Display
  Distance : Scope
  Drag & Friction1 : Subsystem  VariantControl=Choice
  Engine Model : Subsystem
  Gspeed : Scope
  MAP2 : Fcn  Expr=0.98*29.92*(1-u[1]/145442)^5.255876
  Mux4 : Mux  Inputs=3
  OAT2 : Fcn  Expr=(519-0.00357*u[1])-459.67
  RPM : Constant  Value=2000
  Scope1 : Scope
  Sum1 : Sum  Inputs=|++
  Sum2 : Sum  Inputs=+-|
  Terminator : Terminator
  Terminator1 : Terminator
  Terminator2 : Terminator
  Thrust (lb) : Display
  diameter1 : Constant  Value=6.14
  ground speed : Integrator  InitialCondition=20
  headwind : Constant  Value=30
  hp (pressure alt) : Constant  Value=0
  integrator : Integrator
  mu : Constant  Value=.1
  Ft down runway : Outport
  Velocity (ft/s) : Outport  Port=2
  wires:
  [Vtas] -> Mux4/1
  Clo/1 -> Cl Equation/2(Clo)
  Drag & Friction1/1(Drag) -> Sum2/2
  mu/1 -> Drag & Friction1/2(mu)
  Sum1/1 -> [Vtas]  "VTAS"
  AoA (pitch)/1 -> Cl Equation/1(Degrees in)
  COESA Atmosphere Model/3 -> Terminator1/1
  COESA Atmosphere Model/1 -> Terminator/1
  COESA Atmosphere Model/2 -> Terminator2/1
  [Vtas] -> Engine Model/5(In5)
  Sum2/1 -> 1/m/1
  Engine Model/1(Out1) -> Scope1/1, Thrust (lb)/1, Sum2/1
  1/m/1 -> ground speed/1  "xddot"
  Cl Equation/1(Cl) -> Mux4/3, Display/1
  Mux4/1 -> Drag & Friction1/1(Inputs)
  RPM/1 -> [RPM]
  ground speed/1 -> Sum1/1, Velocity (ft/s)/1, Gspeed/1, integrator/1  "xdot"
  hp (pressure alt)/1 -> OAT2/1, MAP2/1, Engine Model/3(In3), COESA Atmosphere Model/1
  MAP2/1 -> Engine Model/1(In1)
  [Diameter] -> Engine Model/6(In6)
  headwind/1 -> Sum1/2
  COESA Atmosphere Model/4 -> Display3/1, Mux4/2
  OAT2/1 -> Engine Model/4(In4)
  [RPM] -> Engine Model/2(In2)
  diameter1/1 -> [Diameter]
  integrator/1 -> Ft down runway/1, Distance/1

== system Takeoff_Sim/groundspeed ==
  x : Inport
  y : Inport  Port=2
  Discrete Derivative : simulink/Discrete/Discrete Derivative  gainval=1.0  ICPrevScaledInput=0.0  OutMin=[]  OutMax=[]  OutDataType=fixdt(1, 16)  OutScaling=2^-10  DoSatur=off
  Discrete Derivative1 : simulink/Discrete/Discrete Derivative  gainval=1.0  ICPrevScaledInput=0.0  OutMin=[]  OutMax=[]  OutDataType=fixdt(1, 16)  OutScaling=2^-10  DoSatur=off
  Sum4 : Sum  Inputs=|++
  Out1 : Outport
  wires:
  Discrete Derivative1/1 -> Sum4/2
  Sum4/1 -> Out1/1
  y/1 -> Discrete Derivative1/1
  x/1 -> Discrete Derivative/1
  Discrete Derivative/1 -> Sum4/1

== system Takeoff_Sim/groundspeed1 ==
  x : Inport
  y : Inport  Port=2
  Discrete Derivative : simulink/Discrete/Discrete Derivative  gainval=1.0  ICPrevScaledInput=0.0  OutMin=[]  OutMax=[]  OutDataType=fixdt(1, 16)  OutScaling=2^-10  DoSatur=off
  Discrete Derivative1 : simulink/Discrete/Discrete Derivative  gainval=1.0  ICPrevScaledInput=0.0  OutMin=[]  OutMax=[]  OutDataType=fixdt(1, 16)  OutScaling=2^-10  DoSatur=off
  Sum4 : Sum  Inputs=|++
  Out1 : Outport
  wires:
  Discrete Derivative1/1 -> Sum4/2
  Sum4/1 -> Out1/1
  y/1 -> Discrete Derivative1/1
  x/1 -> Discrete Derivative/1
  Discrete Derivative/1 -> Sum4/1

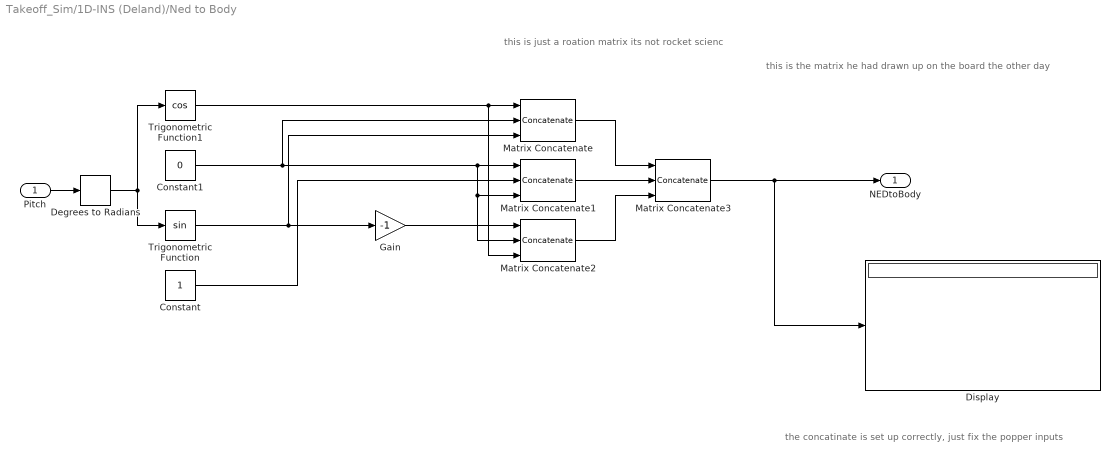
== system Takeoff_Sim/1D-INS (Deland)/Ned to Body ==
  note: this is the matrix he had drawn up on the board the other day
  note: this is just a roation matrix its not rocket scienc
  note: the concatinate is set up correctly, just fix the popper inputs
  Pitch : Inport
  Constant : Constant
  Constant1 : Constant  Value=0
  Degrees to Radians : simulink_extras/Transformations/Degrees to Radians
  Display : Display
  Gain : Gain  Gain=-1
  Matrix Concatenate : Concatenate  NumInputs=3  Mode=Multidimensional array
  Matrix Concatenate1 : Concatenate  NumInputs=3  Mode=Multidimensional array
  Matrix Concatenate2 : Concatenate  NumInputs=3  Mode=Multidimensional array
  Matrix Concatenate3 : Concatenate  NumInputs=3  Mode=Multidimensional array  ConcatenateDimension=2
  Trigonometric Function : Trigonometry
  Trigonometric Function1 : Trigonometry  Operator=cos
  NEDtoBody : Outport
  wires:
  Matrix Concatenate2/1 -> Matrix Concatenate3/3
  Matrix Concatenate/1 -> Matrix Concatenate3/1
  Matrix Concatenate3/1 -> Display/1, NEDtoBody/1
  Matrix Concatenate1/1 -> Matrix Concatenate3/2
  Pitch/1 -> Degrees to Radians/1
  Degrees to Radians/1 -> Trigonometric Function1/1, Trigonometric Function/1
  Trigonometric Function1/1 -> Matrix Concatenate2/3, Matrix Concatenate/1
  Constant1/1 -> Matrix Concatenate2/2, Matrix Concatenate1/3, Matrix Concatenate1/1, Matrix Concatenate/2
  Trigonometric Function/1 -> Gain/1, Matrix Concatenate/3
  Constant/1 -> Matrix Concatenate1/2
  Gain/1 -> Matrix Concatenate2/1

== system Takeoff_Sim/1D-INS (daytona)/Ned to Body ==
  note: this is the matrix he had drawn up on the board the other day
  note: this is just a roation matrix its not rocket scienc
  note: the concatinate is set up correctly, just fix the popper inputs
  Pitch : Inport
  Constant : Constant
  Constant1 : Constant  Value=0
  Degrees to Radians : simulink_extras/Transformations/Degrees to Radians
  Display : Display
  Gain : Gain  Gain=-1
  Matrix Concatenate : Concatenate  NumInputs=3  Mode=Multidimensional array
  Matrix Concatenate1 : Concatenate  NumInputs=3  Mode=Multidimensional array
  Matrix Concatenate2 : Concatenate  NumInputs=3  Mode=Multidimensional array
  Matrix Concatenate3 : Concatenate  NumInputs=3  Mode=Multidimensional array  ConcatenateDimension=2
  Trigonometric Function : Trigonometry
  Trigonometric Function1 : Trigonometry  Operator=cos
  NEDtoBody : Outport
  wires:
  Matrix Concatenate2/1 -> Matrix Concatenate3/3
  Matrix Concatenate/1 -> Matrix Concatenate3/1
  Matrix Concatenate3/1 -> Display/1, NEDtoBody/1
  Matrix Concatenate1/1 -> Matrix Concatenate3/2
  Pitch/1 -> Degrees to Radians/1
  Degrees to Radians/1 -> Trigonometric Function1/1, Trigonometric Function/1
  Trigonometric Function1/1 -> Matrix Concatenate2/3, Matrix Concatenate/1
  Constant1/1 -> Matrix Concatenate2/2, Matrix Concatenate1/3, Matrix Concatenate1/1, Matrix Concatenate/2
  Trigonometric Function/1 -> Gain/1, Matrix Concatenate/3
  Constant/1 -> Matrix Concatenate1/2
  Gain/1 -> Matrix Concatenate2/1

== system Takeoff_Sim/Physics Based System (Deland)/Cl Equation ==
  note: on flat runway theta=AoA, then Cl=Cl_alpha*alpha, which should e a constant, and it should probably be zero, if there is no AoA, I would only try with nonzero
  note: go to aero text book and figure out CL_alpha based on the aspect ratio of that airplane in incompressible flow.
  Degrees in : Inport
  Clo : Inport  Port=2
  CLa : Constant  Value=2*pi/(1+2/(e*AR))
  Degrees to Radians : simulink_extras/Transformations/Degrees to Radians
  Display : Display
  Product : Product
  Sum3 : Sum  Inputs=|++
  Cl : Outport
  wires:
  CLa/1 -> Display/1, Product/2
  Sum3/1 -> Cl/1
  Degrees to Radians/1 -> Product/1
  Degrees in/1 -> Degrees to Radians/1
  Clo/1 -> Sum3/2
  Product/1 -> Sum3/1

== system Takeoff_Sim/Physics Based System (Deland)/Drag & Friction1 ==
  note: weight minus lift times rolling friction coef which we can pull from our book
  Inputs : Inport
  mu : Inport  Port=2
  Gain2 : Gain
  Induced Drag : Fcn  Expr=0.5 * u[2] * u[1]^2 * S * u[3]^2 / (3.14 * e * AR)
  Mux : Mux  Inputs=2
  Parasite Drag : Fcn  Expr=0.5*u[2]*u[1]^2*f
  Saturation : Saturate  UpperLimit=1000  LowerLimit=0
  Scope3 : Scope  NumInputPorts=3
  Sum : Sum  Inputs=+++
  friction : Fcn  Expr=u[4] * (Weight - 0.5 * u[2] * u[1]^2 * S * u[3])
  lift : Fcn  Expr=0.5 * u[2] * u[1]^2 * S * u[3]
  lift (lbs) : Scope
  Drag : Outport
  wires:
  mu/1 -> Mux/2
  Sum/1 -> Drag/1
  lift/1 -> lift (lbs)/1
  Mux/1 -> friction/1, lift/1
  Gain2/1 -> Sum/2, Scope3/2  "induced"
  Parasite Drag/1 -> Sum/1, Scope3/1  "parasite"
  Induced Drag/1 -> Gain2/1
  Inputs/1 -> Induced Drag/1, Mux/1, Parasite Drag/1
  friction/1 -> Saturation/1
  Saturation/1 -> Sum/3, Scope3/3  "friction"

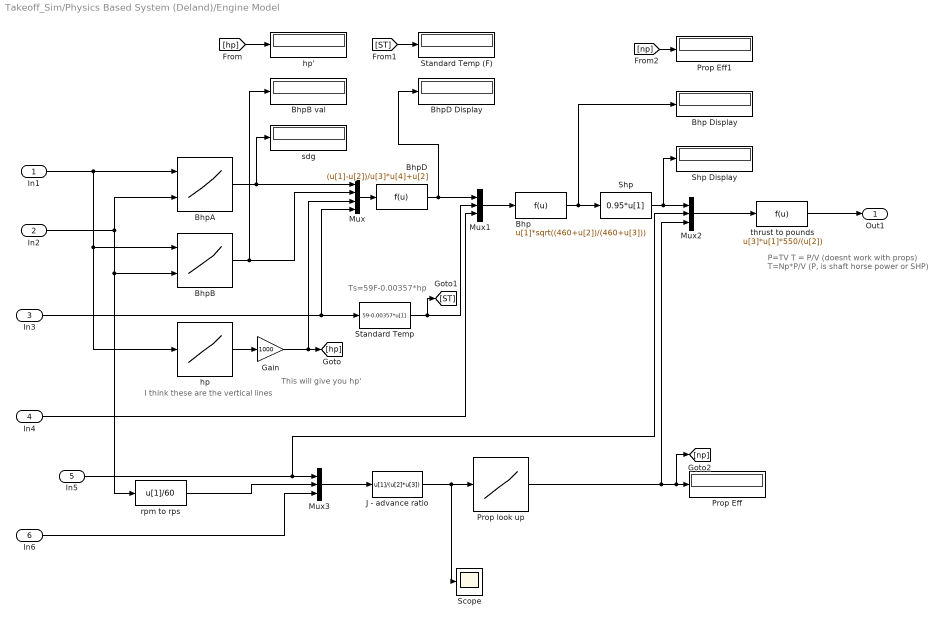
== system Takeoff_Sim/Physics Based System (Deland)/Engine Model ==
  note: This will give you hp'
  note: P=TV
      |
      | T = P/V (doesnt work with props)
      | T=Np*P/V (P, is shaft horse power or SHP)
  note: Ts=59F-0.00357*hp
  note: I think these are the vertical lines
  In1 : Inport
  In2 : Inport  Port=2
  In3 : Inport  Port=3
  In4 : Inport  Port=4
  In5 : Inport  Port=5
  In6 : Inport  Port=6
  Bhp : Fcn  Expr=u[1]*sqrt((460+u[2])/(460+u[3]))
  Bhp Display : Display
  BhpA : Lookup_n-D  BreakpointsForDimension1=[12;14;16;18;20;22;24;26;28]  BreakpointsForDimension2=[2000 2200 2400 2600 2700]  Table=[55 65 68 70 71;69 77 82 84 87;79 87 94 97 100;88 98 105 111 115;98 108 116 123 126;108 119 127 135 140;119 129 138 147 153;127 139 150 160 164;138 149 161 172 177]  InternalRulePriority=Speed  RndMeth=Simplest
      settings: InputPortMap=u0,u1
  BhpB : Lookup_n-D  BreakpointsForDimension1=[17 18 19 20 21 22 23 24 25 26 27 28 29]  BreakpointsForDimension2=[2000 2200 2400 2600 2700]  Table=[60 68 71 81 82;65 74 80 98 90;73 81 86 95 98;80 87 94 103 106;85 95 102 111 116;93 103 110 120 123;100 110 118 126 133;106 115 125 135 141;116 124 135 144 150;120 131 143 152 158;125 137 148 159 165;135 145 157 167 173;142 153 165 176 183]  InternalRulePriority=Speed  RndMeth=Simplest
      settings: InputPortMap=u0,u1
  BhpB val : Display
  BhpD : Fcn  Expr=(u[1]-u[2])/u[3]*u[4]+u[2]
  BhpD Display : Display
  Gain : Gain  Gain=1000
  J - advance ratio : Fcn  Expr=u[1]/(u[2]*u[3])
  Mux : Mux
  Mux1 : Mux  Inputs=3
  Mux2 : Mux  Inputs=3
  Mux3 : Mux  Inputs=3
  Prop Eff : Display
  Prop Eff1 : Display
  Prop look up : Lookup_n-D  NumberOfTableDimensions=1  BreakpointsForDimension1=[0;0.048012249;0.060807878;0.079983697;0.105563205;0.133281193;0.157430152;0.178753263;0.199368443;0.215001671;0.227800237;0.245557257;0.273971426;0.300949171;0.327207235;0.352754431;0.371192944;0.390339388;0.409494645;0.433608354;0.457002383;0.472603298;0.491041811;0.509471512;0.534281402;0.552003172;0.576810125;0.598782418;0.619332973;0.645549913;0.671763915;0.690895672;0.717103799;0.745432781;0.760302266;0.778708467;0.799946391;0.819051711;0.845926644;0.867848999;0.888343743;0.903180915;0.92013013;0.934250559;0.947645432;0.961736487;0.970184657;0.980736057;0.986337817;0.992650444;0.994753675]  Table=[0;0.109900628;0.134509301;0.163123953;0.206809061;0.257361734;0.294163365;0.333794761;0.373442069;0.400753217;0.42674495;0.454008364;0.499012887;0.534367813;0.564206411;0.592677861;0.607477825;0.622261878;0.641195111;0.661400024;0.676088609;0.688186099;0.702986063;0.713636848;0.72829361;0.738960306;0.752234009;0.764188297;0.773408288;0.783884048;0.792976749;0.800845502;0.807172083;0.81206787;0.813116793;0.812703099;0.812225759;0.807646975;0.794594806;0.783037077;0.765978931;0.751814195;0.732069486;0.713771482;0.68719103;0.655062427;0.632742534;0.600693488;0.571521941;0.543717542;0.53398839]  InternalRulePriority=Speed  RndMeth=Simplest
  Scope : Scope
  Shp : Fcn  Expr=0.95*u[1]
  Shp Display : Display
  Standard Temp : Fcn  Expr=59-0.00357*u[1]
  Standard Temp (F) : Display
  hp : Lookup_n-D  NumberOfTableDimensions=1  BreakpointsForDimension1=[12, 14, 16, 18, 20, 22, 24, 26, 28]  Table=[22.5, 19.3, 15.8, 12.8, 10.3, 7.8, 5.5, 3.25, 1.4]  InternalRulePriority=Speed  RndMeth=Simplest
  "hp' " : Display
  rpm to rps : Fcn  Expr=u[1]/60
  sdg : Display
  thrust to pounds : Fcn  Expr=u[3]*u[1]*550/(u[2])
  Out1 : Outport
  wires:
  In6/1 -> Mux3/3
  In4/1 -> Mux1/3
  BhpA/1 -> Mux/1, sdg/1
  BhpD/1 -> Mux1/1, BhpD Display/1
  Mux2/1 -> thrust to pounds/1
  In5/1 -> Mux3/1, Mux2/2
  Bhp/1 -> Shp/1, Bhp Display/1
  thrust to pounds/1 -> Out1/1
  In3/1 -> Standard Temp/1, Mux/4
  Standard Temp/1 -> Mux1/2, [ST]
  BhpB/1 -> Mux/2, BhpB val/1
  Mux1/1 -> Bhp/1
  In2/1 -> rpm to rps/1, BhpB/2, BhpA/2
  In1/1 -> BhpA/1, BhpB/1, hp/1
  Shp/1 -> Mux2/1, Shp Display/1
  [np] -> Prop Eff1/1
  J - advance ratio/1 -> Prop look up/1, Scope/1
  Prop look up/1 -> Mux2/3, Prop Eff/1, [np]
  Mux/1 -> BhpD/1
  rpm to rps/1 -> Mux3/2
  [hp] -> "hp' "/1
  Mux3/1 -> J - advance ratio/1
  [ST] -> Standard Temp (F)/1
  Gain/1 -> Mux/3, [hp]
  hp/1 -> Gain/1

== system Takeoff_Sim/Physics Based System (daytona)/Cl Equation ==
  note: go to aero text book and figure out CL_alpha based on the aspect ratio of that airplane in incompressible flow.
  note: on flat runway theta=AoA, then Cl=Cl_alpha*alpha, which should e a constant, and it should probably be zero, if there is no AoA, I would only try with nonzero
  Degrees in : Inport
  Clo : Inport  Port=2
  CLa : Constant  Value=2*pi/(1+2/(e*AR))
  Degrees to Radians : simulink_extras/Transformations/Degrees to Radians
  Display : Display
  Product : Product
  Sum3 : Sum  Inputs=|++
  Cl : Outport
  wires:
  Product/1 -> Sum3/1
  Clo/1 -> Sum3/2
  Degrees in/1 -> Degrees to Radians/1
  Degrees to Radians/1 -> Product/1
  Sum3/1 -> Cl/1
  CLa/1 -> Product/2, Display/1

== system Takeoff_Sim/Physics Based System (daytona)/Drag & Friction1 ==
  note: weight minus lift times rolling friction coef which we can pull from our book
  Inputs : Inport
  mu : Inport  Port=2
  Gain2 : Gain
  Induced Drag : Fcn  Expr=0.5 * u[2] * u[1]^2 * S * u[3]^2 / (3.14 * e * AR)
  Mux : Mux  Inputs=2
  Parasite Drag : Fcn  Expr=0.5*u[2]*u[1]^2*f
  Saturation : Saturate  UpperLimit=1000  LowerLimit=0
  Scope3 : Scope  NumInputPorts=3
  Sum : Sum  Inputs=+++
  friction : Fcn  Expr=u[4] * (Weight - 0.5 * u[2] * u[1]^2 * S * u[3])
  lift : Fcn  Expr=0.5 * u[2] * u[1]^2 * S * u[3]
  lift (lbs) : Scope
  Drag : Outport
  wires:
  Saturation/1 -> Scope3/3, Sum/3  "friction"
  friction/1 -> Saturation/1
  Inputs/1 -> Parasite Drag/1, Mux/1, Induced Drag/1
  Induced Drag/1 -> Gain2/1
  Parasite Drag/1 -> Scope3/1, Sum/1  "parasite"
  Gain2/1 -> Scope3/2, Sum/2  "induced"
  Mux/1 -> lift/1, friction/1
  lift/1 -> lift (lbs)/1
  Sum/1 -> Drag/1
  mu/1 -> Mux/2

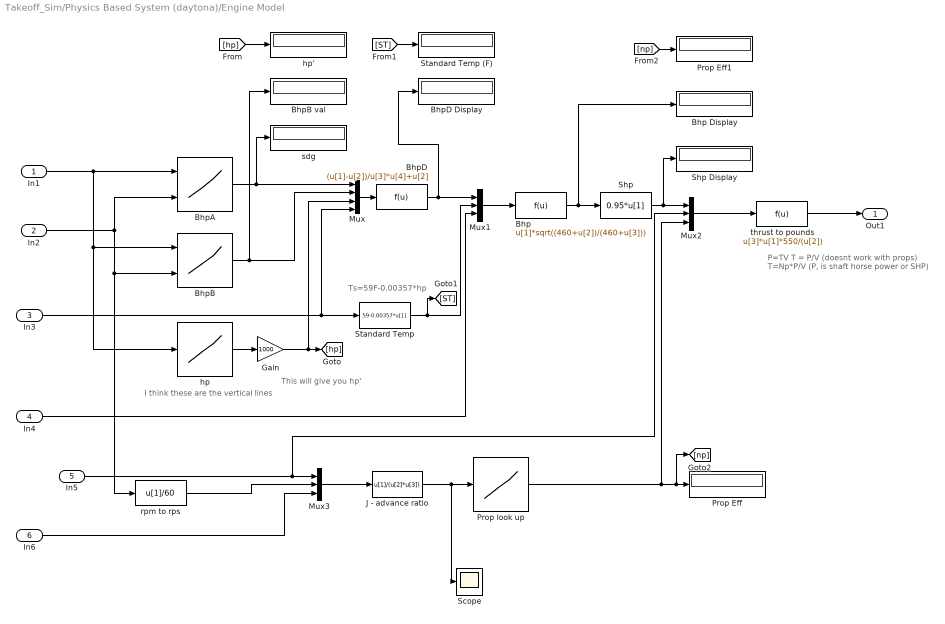
== system Takeoff_Sim/Physics Based System (daytona)/Engine Model ==
  note: I think these are the vertical lines
  note: Ts=59F-0.00357*hp
  note: P=TV
      |
      | T = P/V (doesnt work with props)
      | T=Np*P/V (P, is shaft horse power or SHP)
  note: This will give you hp'
  In1 : Inport
  In2 : Inport  Port=2
  In3 : Inport  Port=3
  In4 : Inport  Port=4
  In5 : Inport  Port=5
  In6 : Inport  Port=6
  Bhp : Fcn  Expr=u[1]*sqrt((460+u[2])/(460+u[3]))
  Bhp Display : Display
  BhpA : Lookup_n-D  BreakpointsForDimension1=[12;14;16;18;20;22;24;26;28]  BreakpointsForDimension2=[2000 2200 2400 2600 2700]  Table=[55 65 68 70 71;69 77 82 84 87;79 87 94 97 100;88 98 105 111 115;98 108 116 123 126;108 119 127 135 140;119 129 138 147 153;127 139 150 160 164;138 149 161 172 177]  InternalRulePriority=Speed  RndMeth=Simplest
      settings: InputPortMap=u0,u1
  BhpB : Lookup_n-D  BreakpointsForDimension1=[17 18 19 20 21 22 23 24 25 26 27 28 29]  BreakpointsForDimension2=[2000 2200 2400 2600 2700]  Table=[60 68 71 81 82;65 74 80 98 90;73 81 86 95 98;80 87 94 103 106;85 95 102 111 116;93 103 110 120 123;100 110 118 126 133;106 115 125 135 141;116 124 135 144 150;120 131 143 152 158;125 137 148 159 165;135 145 157 167 173;142 153 165 176 183]  InternalRulePriority=Speed  RndMeth=Simplest
      settings: InputPortMap=u0,u1
  BhpB val : Display
  BhpD : Fcn  Expr=(u[1]-u[2])/u[3]*u[4]+u[2]
  BhpD Display : Display
  Gain : Gain  Gain=1000
  J - advance ratio : Fcn  Expr=u[1]/(u[2]*u[3])
  Mux : Mux
  Mux1 : Mux  Inputs=3
  Mux2 : Mux  Inputs=3
  Mux3 : Mux  Inputs=3
  Prop Eff : Display
  Prop Eff1 : Display
  Prop look up : Lookup_n-D  NumberOfTableDimensions=1  BreakpointsForDimension1=[0;0.048012249;0.060807878;0.079983697;0.105563205;0.133281193;0.157430152;0.178753263;0.199368443;0.215001671;0.227800237;0.245557257;0.273971426;0.300949171;0.327207235;0.352754431;0.371192944;0.390339388;0.409494645;0.433608354;0.457002383;0.472603298;0.491041811;0.509471512;0.534281402;0.552003172;0.576810125;0.598782418;0.619332973;0.645549913;0.671763915;0.690895672;0.717103799;0.745432781;0.760302266;0.778708467;0.799946391;0.819051711;0.845926644;0.867848999;0.888343743;0.903180915;0.92013013;0.934250559;0.947645432;0.961736487;0.970184657;0.980736057;0.986337817;0.992650444;0.994753675]  Table=[0;0.109900628;0.134509301;0.163123953;0.206809061;0.257361734;0.294163365;0.333794761;0.373442069;0.400753217;0.42674495;0.454008364;0.499012887;0.534367813;0.564206411;0.592677861;0.607477825;0.622261878;0.641195111;0.661400024;0.676088609;0.688186099;0.702986063;0.713636848;0.72829361;0.738960306;0.752234009;0.764188297;0.773408288;0.783884048;0.792976749;0.800845502;0.807172083;0.81206787;0.813116793;0.812703099;0.812225759;0.807646975;0.794594806;0.783037077;0.765978931;0.751814195;0.732069486;0.713771482;0.68719103;0.655062427;0.632742534;0.600693488;0.571521941;0.543717542;0.53398839]  InternalRulePriority=Speed  RndMeth=Simplest
  Scope : Scope
  Shp : Fcn  Expr=0.95*u[1]
  Shp Display : Display
  Standard Temp : Fcn  Expr=59-0.00357*u[1]
  Standard Temp (F) : Display
  hp : Lookup_n-D  NumberOfTableDimensions=1  BreakpointsForDimension1=[12, 14, 16, 18, 20, 22, 24, 26, 28]  Table=[22.5, 19.3, 15.8, 12.8, 10.3, 7.8, 5.5, 3.25, 1.4]  InternalRulePriority=Speed  RndMeth=Simplest
  "hp' " : Display
  rpm to rps : Fcn  Expr=u[1]/60
  sdg : Display
  thrust to pounds : Fcn  Expr=u[3]*u[1]*550/(u[2])
  Out1 : Outport
  wires:
  hp/1 -> Gain/1
  Gain/1 -> [hp], Mux/3
  [ST] -> Standard Temp (F)/1
  Mux3/1 -> J - advance ratio/1
  [hp] -> "hp' "/1
  rpm to rps/1 -> Mux3/2
  Mux/1 -> BhpD/1
  Prop look up/1 -> [np], Prop Eff/1, Mux2/3
  J - advance ratio/1 -> Scope/1, Prop look up/1
  [np] -> Prop Eff1/1
  Shp/1 -> Shp Display/1, Mux2/1
  In1/1 -> hp/1, BhpB/1, BhpA/1
  In2/1 -> BhpA/2, BhpB/2, rpm to rps/1
  Mux1/1 -> Bhp/1
  BhpB/1 -> BhpB val/1, Mux/2
  Standard Temp/1 -> [ST], Mux1/2
  In3/1 -> Mux/4, Standard Temp/1
  thrust to pounds/1 -> Out1/1
  Bhp/1 -> Bhp Display/1, Shp/1
  In5/1 -> Mux2/2, Mux3/1
  Mux2/1 -> thrust to pounds/1
  BhpD/1 -> BhpD Display/1, Mux1/1
  BhpA/1 -> sdg/1, Mux/1
  In4/1 -> Mux1/3
  In6/1 -> Mux3/3
